simulink model "Servo_LQ_D_sim"  (R2022b)
settings: Solver=ode5  StartTime=0.0  StopTime=5  FixedStep=T0  RelTol=1e-3  AbsTol=1e-6
values from neighbouring files (symbols this model uses):
  K = [0.06  0.0 0.0125]    [servo_start.m]
  Ks = 195    [Servo_calc_lq.m]    (also in Servo_calc_lq_d.m; servo_start.m)
  T0 = 0.01    [Servo_calc_lq.m]    (also in Servo_calc_lq_d.m; servo_start.m = 0.1)
  Ts = 0.86    [Servo_calc_lq.m]    (also in Servo_calc_lq_d.m; servo_start.m)
settings Model: ExtModeTrigDuration=20000  ExtModeTrigLevel=0.400000  Creator=jims  LastModifiedBy=artur
settings SolverCC: AutoScaleAbsTol=off  AlgebraicLoopSolver=TrustRegion
settings DataIOCC: ExternalInput=[]  InitialState=[]  MaxDataPoints=5000  SaveFormat=Array  SignalLoggingSaveFormat=ModelDataLogs  SaveOutput=off  SaveTime=off  ReturnWorkspaceOutputs=off  SignalLoggingName=sigsOut
settings OptimizationCC: BooleanDataType=off  ExpressionDepthLimit=2147483647  LifeSpan=inf
settings DebuggingCC: SaveWithParameterizedLinksMsg=none  UnderspecifiedInitializationDetection=Classic  MergeDetectMultiDrivingBlocksExec=none  SignalResolutionControl=TryResolveAllWithWarning  MultiTaskDSMMsg=warning  MultiTaskCondExecSysMsg=none  IntegerOverflowMsg=none  FcnCallInpInsideContextMsg=warning  UnconnectedInputMsg=warning  UnconnectedOutputMsg=warning  UnconnectedLineMsg=warning  StateNameClashWarn=warning  SFUnexpectedBacktrackingDiag=warning  SFNoUnconditionalDefaultTransitionDiag=warning  SFExecutionAtInitializationDiag=none  SFMachineParentedDataDiag=warning  IntegerSaturationMsg=none  ArithmeticOperatorsInVariantConditions=warning
settings HardwareCC: ProdBitPerPointer=32  ProdBitPerSizeT=32  ProdBitPerPtrDiffT=32  ProdLargestAtomicFloat=None  ProdWordSize=32  ProdHWDeviceType=Generic->32-bit x86 compatible  TargetBitPerPointer=64  TargetBitPerSizeT=64  TargetBitPerPtrDiffT=64  TargetLongLongMode=on  TargetIntDivRoundTo=Zero  TargetEndianess=LittleEndian  TargetWordSize=64  TargetHWDeviceType=MATLAB Host  ProdEqTarget=off
settings ModelReferenceCC: EnableRefExpFcnMdlSchedulingChecks=on  PropagateSignalLabelsOutOfModel=off
settings SFSimCC: SimUseLocalCustomCode=off  CustomCodeUndefinedFunction=UseInterfaceOnly
settings RTWCC: Description=servo (Visual C/C++)  SystemTargetFile=rtcon_servo_USB2.tlc  TemplateMakefile=servo_vc_USB2_x64.tmf  RTWUseLocalCustomCode=off  RTWCompilerOptimization=on
settings CodeAppCC: StateflowObjectComments=on
settings STFCustomTargetCC: ModelReferenceCompliant=off  CombineOutputUpdateFcns=on  MatFileLogging=on  CPPClassGenCompliant=on  SystemTargetFile=rtcon_servo_USB2.tlc
settings GRTTargetCC: TargetLangStandard=C89/C90 (ANSI)  ModelReferenceCompliant=off  ParMdlRefBuildCompliant=off  CompOptLevelCompliant=off  ConcurrentExecutionCompliant=off  UseToolchainInfoCompliant=off
settings ConfigComp: CovMetricSettings=dw  CovSaveCumulativeToWorkspaceVar=on  CovSaveSingleToWorkspaceVar=on  CovExternalEMLEnable=off  CovSFcnEnable=off

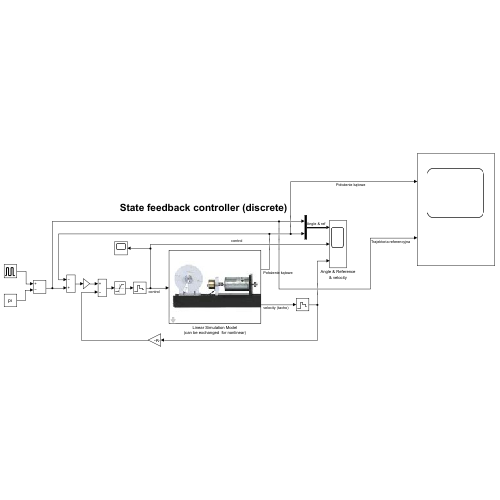
[thumbnail: Simulink's stored preview of the top-level diagram]
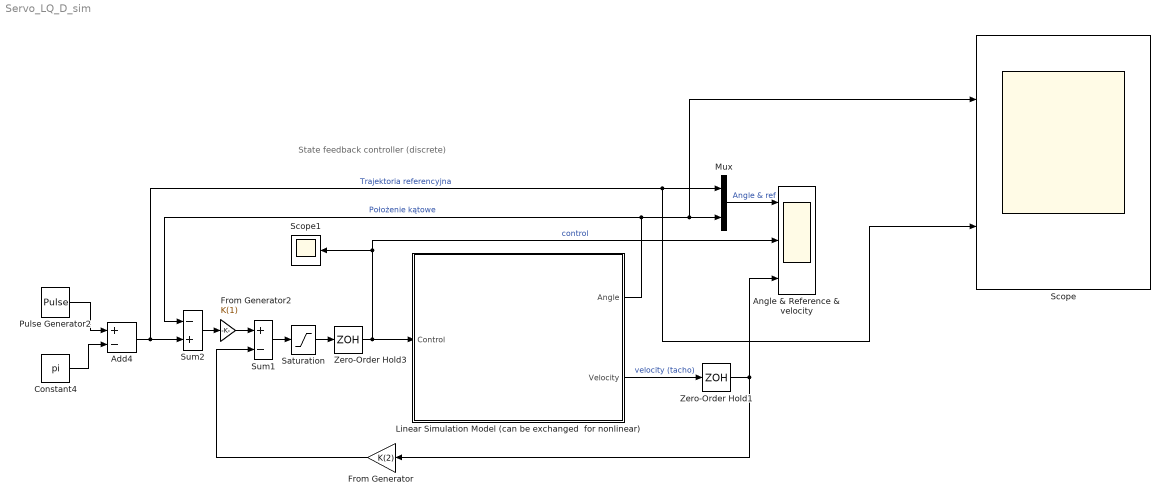
== system Servo_LQ_D_sim ==
  note: State feedback controller (discrete)
  Add4 : Sum  Inputs=+-
  Angle & Reference & velocity : Scope  NumInputPorts=3
  Constant4 : Constant  Value=pi
  From Generator : Gain  Gain=K(2)  SaturateOnIntegerOverflow=on  OutDataTypeStr=Inherit: Same as input  ParamDataTypeStr=Inherit: Same as input
  From Generator2 : Gain  Gain=K(1)  SaturateOnIntegerOverflow=on  OutDataTypeStr=Inherit: Same as input  ParamDataTypeStr=Inherit: Same as input
  Linear Simulation Model (can be exchanged  for nonlinear) : Subsystem  mask{x0=[0 0]}
      mask prompts: x0 "Initial conditions [angle vel]"
      mask Display: image(imread('Servo_m.JPG'))
  Mux : Mux  Inputs=2
  Pulse Generator2 : DiscretePulseGenerator  PulseType=Time based  Amplitude=2*pi  Period=4  PulseWidth=50
  Saturation : Saturate  UpperLimit=1  LowerLimit=-1
  Scope : Scope  NumInputPorts=2
  Scope1 : Scope
  Sum1 : Sum  Inputs=+-  InputSameDT=on  SaturateOnIntegerOverflow=on  OutDataTypeStr=Inherit: Same as first input
  Sum2 : Sum  Inputs=-+  InputSameDT=on  SaturateOnIntegerOverflow=on  OutDataTypeStr=Inherit: Same as first input
  Zero-Order Hold1 : ZeroOrderHold  SampleTime=T0
  Zero-Order Hold3 : ZeroOrderHold  SampleTime=T0
  wires:
  Mux/1 -> Angle & Reference & velocity/1  "Angle & ref"
  Linear Simulation Model (can be exchanged  for nonlinear)/1(Angle) -> Scope/1, Mux/2, Sum2/1  "Położenie kątowe"
  Linear Simulation Model (can be exchanged  for nonlinear)/2(Velocity) -> Zero-Order Hold1/1  "velocity (tacho)"
  Add4/1 -> Sum2/2, Scope/2, Mux/1  "Trajektoria referencyjna"
  Sum1/1 -> Saturation/1
  From Generator2/1 -> Sum1/1
  From Generator/1 -> Sum1/2
  Saturation/1 -> Zero-Order Hold3/1
  Zero-Order Hold3/1 -> Scope1/1, Angle & Reference & velocity/2, Linear Simulation Model (can be exchanged  for nonlinear)/1(Control)  "control"
  Sum2/1 -> From Generator2/1
  Zero-Order Hold1/1 -> Angle & Reference & velocity/3, From Generator/1
  Constant4/1 -> Add4/2
  Pulse Generator2/1 -> Add4/1

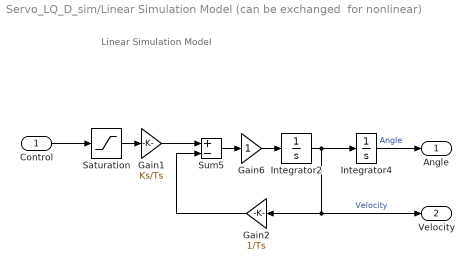
== system Servo_LQ_D_sim/Linear Simulation Model (can be exchanged  for nonlinear) ==
  note: Linear Simulation Model
  Control : Inport
  Gain1 : Gain  Gain=Ks/Ts  SaturateOnIntegerOverflow=on  OutDataTypeStr=Inherit: Same as input  ParamDataTypeStr=Inherit: Same as input
  Gain2 : Gain  Gain=1/Ts  SaturateOnIntegerOverflow=on  OutDataTypeStr=Inherit: Same as input  ParamDataTypeStr=Inherit: Same as input
  Gain6 : Gain  SaturateOnIntegerOverflow=on  OutDataTypeStr=Inherit: Same as input  ParamDataTypeStr=Inherit: Same as input
  Integrator2 : Integrator  InitialCondition=x0(2)
  Integrator4 : Integrator  InitialCondition=x0(1)
  Saturation : Saturate  UpperLimit=1  LowerLimit=-1
  Sum5 : Sum  Inputs=+-  InputSameDT=on  SaturateOnIntegerOverflow=on  OutDataTypeStr=Inherit: Same as first input
  Angle : Outport  InitialOutput=0  VectorParamsAs1DForOutWhenUnconnected=off
  Velocity : Outport  Port=2  InitialOutput=0  VectorParamsAs1DForOutWhenUnconnected=off
  wires:
  Gain1/1 -> Sum5/1
  Saturation/1 -> Gain1/1
  Control/1 -> Saturation/1
  Gain6/1 -> Integrator2/1
  Integrator4/1 -> Angle/1  "Angle"
  Integrator2/1 -> Gain2/1, Velocity/1, Integrator4/1  "Velocity"
  Gain2/1 -> Sum5/2
  Sum5/1 -> Gain6/1
